simulink model "DriveTrain_SystemID3"  (R2019a)
settings: Solver=VariableStepAuto  StartTime=0.0  StopTime=20  MaxStep=1e-3  RelTol=1e-3
InitFcn:
  | %DriveTrainInitialise;
values from neighbouring files (symbols this model uses):
  D = 0.04925    [DrivetrainParametersForRhys.m]
  J = 0.0256    [DrivetrainParametersForRhys.m]
  Ld = 125e-6    (= 0.000125)    [DrivetrainParametersForRhys.m]
  Lq = 130e-6    (= 0.00013)    [DrivetrainParametersForRhys.m]
  p = PolePairs    (= 10)    [DrivetrainParametersForRhys.m]
  PM = 0.0393    [DrivetrainParametersForRhys.m]
  rate = 20    [DrivetrainParametersForRhys.m]
  ratio = 3.27    [DrivetrainParametersForRhys.m]
  Rs = 0.35    [DrivetrainParametersForRhys.m]
  Ts = 1/fs    (= 8.33333333333e-06)    [DrivetrainParametersForRhys.m]    (also in GreyBoxSystemID.m = mean(diff(posTime)))
  Tsc = 1/fc    (= 0.000166666666667)    [DrivetrainParametersForRhys.m]
  Vnom = 450    [DrivetrainParametersForRhys.m]
undefined symbols (not defined in the file or in its folder): Iq_max, Kaw, kdI, kdP, Ki, Kp, kqI, kqP
libraries: eeDqVoltageLimiter x1, eeTransforms x1
settings Model: OrderedModelArguments=off  Creator=plewi  LastModifiedBy=plewi

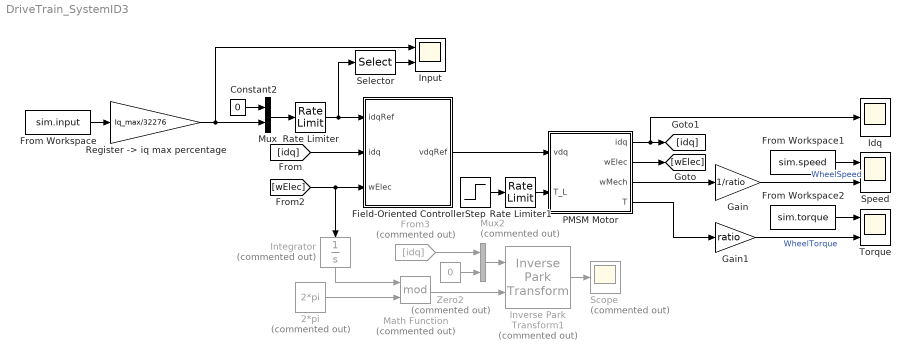
== system DriveTrain_SystemID3 ==
  2*pi : Constant  Commented=on  Value=2*pi  SampleTime=Tsc
  Constant2 : Constant  Value=0
  Field-Oriented Controller : Subsystem
  From Workspace : FromWorkspace  VariableName=sim.input  SampleTime=0
  From Workspace1 : FromWorkspace  VariableName=sim.speed  SampleTime=0
  From Workspace2 : FromWorkspace  VariableName=sim.torque  SampleTime=0
  From3 : From  Commented=on  GotoTag=idq
  Gain : Gain  Gain=1/ratio
  Gain1 : Gain  Gain=ratio
  Idq : Scope
  Input : Scope  NumInputPorts=2
  Integrator : Integrator  Commented=on
  Inverse Park Transform1 : eeTransforms/Inverse Park Transform  Commented=on  AxisAlignment=Q-axis  PowerInvariant=off
      settings: SourceProductName=Simscape Electrical
  Math Function : Math  Commented=on  Operator=mod  SaturateOnIntegerOverflow=on
  Mux : Mux  Inputs=2
  Mux2 : Mux  Commented=on  Inputs=2
  PMSM Motor : Subsystem
  Rate Limiter : RateLimiter  RisingSlewLimit=rate  FallingSlewLimit=-rate  SampleTimeMode=inherited
  Rate Limiter1 : RateLimiter  RisingSlewLimit=rate  FallingSlewLimit=-rate  SampleTimeMode=inherited
  "Register -> iq max percentage" : Gain  Gain=Iq_max/32276
  Scope : Scope  Commented=on
  Selector : Selector  InputPortWidth=2  IndexOptions=Index vector (dialog)  Indices=[2]  OutputSizes=1
  Speed : Scope  NumInputPorts=2
  Step : Step  Time=0  After=0  SampleTime=0
  Torque : Scope  NumInputPorts=2
  Zero2 : Constant  Commented=on  Value=0  OutDataTypeStr=Inherit: Inherit via back propagation
  wires:
  From Workspace/1 -> "Register -> iq max percentage"/1
  "Register -> iq max percentage"/1 -> Input/1, Mux/2
  Constant2/1 -> Mux/1
  From Workspace1/1 -> Speed/1
  From Workspace2/1 -> Torque/1
  Mux/1 -> Rate Limiter/1
  Rate Limiter/1 -> Selector/1, Field-Oriented Controller/1(idqRef)
  Selector/1 -> Input/2
  2*pi/1 -> Math Function/2
  Integrator/1 -> Math Function/1
  [wElec] -> Field-Oriented Controller/3(wElec), Integrator/1
  PMSM Motor/1("idq ") -> Idq/1, [idq]
  [idq] -> Field-Oriented Controller/2(idq)
  PMSM Motor/2(wElec) -> [wElec]
  Gain/1 -> Speed/2  "WheelSpeed"
  PMSM Motor/3(wMech) -> Gain/1
  PMSM Motor/4(T) -> Gain1/1
  Gain1/1 -> Torque/2  "WheelTorque"
  Math Function/1 -> Inverse Park Transform1/2
  Inverse Park Transform1/1 -> Scope/1
  Zero2/1 -> Mux2/2
  From3/1 -> Mux2/1
  Mux2/1 -> Inverse Park Transform1/1
  Field-Oriented Controller/1(vdqRef) -> PMSM Motor/1(vdq)
  Step/1 -> Rate Limiter1/1
  Rate Limiter1/1 -> PMSM Motor/2(T_L)

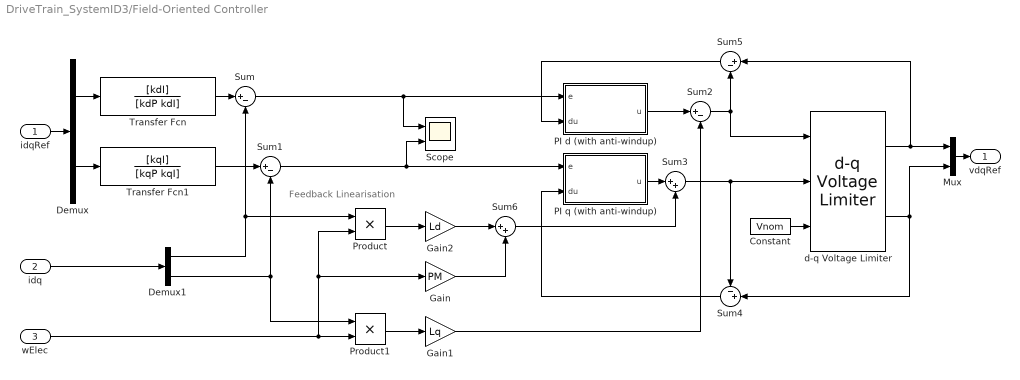
== system DriveTrain_SystemID3/Field-Oriented Controller ==
  note: Feedback Linearisation
  idqRef : Inport  SampleTime=Ts
  idq : Inport  Port=2  SampleTime=Ts
  wElec : Inport  Port=3  SampleTime=Ts
  Constant : Constant  Value=Vnom
  Demux : Demux  Outputs=2
  Demux1 : Demux  Outputs=2
  Gain : Gain  Gain=PM
  Gain1 : Gain  Gain=Lq
  Gain2 : Gain  Gain=Ld
  Mux : Mux  Inputs=2
  PI d (with anti-windup) : Subsystem
  PI q (with anti-windup) : Subsystem
  Product : Product
  Product1 : Product
  Scope : Scope  NumInputPorts=2
  Sum{,1..2,5} (4 alike) : Sum  Inputs=|+-
  Sum3 : Sum  Inputs=|++
  Sum4 : Sum  Inputs=-+|
  Sum6 : Sum  Inputs=|++
  Transfer Fcn : TransferFcn  Numerator=[kdI]  Denominator=[kdP kdI]
  Transfer Fcn1 : TransferFcn  Numerator=[kqI]  Denominator=[kqP kqI]
  d-q Voltage Limiter : eeDqVoltageLimiter/d-q Voltage Limiter  AxisPrio=Q-axis  Ts=-1
      settings: SourceProductName=Simscape Electrical  SourceProductBaseCode=PS
  vdqRef : Outport
  wires:
  Sum/1 -> Scope/1, PI d (with anti-windup)/1(e)
  Transfer Fcn1/1 -> Sum1/1
  Transfer Fcn/1 -> Sum/1
  d-q Voltage Limiter/2 -> Mux/2, Sum4/2
  idq/1 -> Demux1/1
  idqRef/1 -> Demux/1
  Sum2/1 -> d-q Voltage Limiter/1, Sum5/2
  Sum5/1 -> PI d (with anti-windup)/2(du)
  Demux/1 -> Transfer Fcn/1
  Constant/1 -> d-q Voltage Limiter/3
  Demux/2 -> Transfer Fcn1/1
  Sum3/1 -> d-q Voltage Limiter/2, Sum4/1
  d-q Voltage Limiter/1 -> Mux/1, Sum5/1
  Sum6/1 -> Sum3/2
  PI d (with anti-windup)/1(u) -> Sum2/1
  Sum4/1 -> PI q (with anti-windup)/2(du)
  Sum1/1 -> Scope/2, PI q (with anti-windup)/1(e)
  PI q (with anti-windup)/1(u) -> Sum3/1
  Demux1/1 -> Product/1, Sum/2
  Demux1/2 -> Sum1/2, Product1/1
  Gain/1 -> Sum6/2
  Product1/1 -> Gain1/1
  Gain1/1 -> Sum2/2
  Product/1 -> Gain2/1
  Gain2/1 -> Sum6/1
  wElec/1 -> Gain/1, Product/2, Product1/2
  Mux/1 -> vdqRef/1

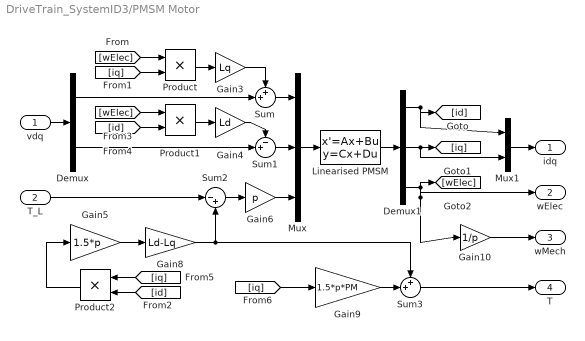
== system DriveTrain_SystemID3/PMSM Motor ==
  vdq : Inport
  T_L : Inport  Port=2
  Demux : Demux  Outputs=2
  Demux1 : Demux  Outputs=3
  Gain10 : Gain  Gain=1/p
  Gain3 : Gain  Gain=Lq
  Gain4 : Gain  Gain=Ld
  Gain5 : Gain  Gain=1.5*p
  Gain6 : Gain  Gain=p
  Gain8 : Gain  Gain=Ld-Lq
  Gain9 : Gain  Gain=1.5*p*PM
  "Linearised PMSM " : StateSpace  A=inv(diag([Ld,Lq,J]))*[-Rs, 0, 0; 0, -Rs, -PM; 0, 1.5*(p^2)*PM, -D]  B=inv(diag([Ld,Lq,J]))*eye(3)  C=eye(3)  D=zeros(3)  InitialCondition=0
  Mux : Mux  Inputs=3
  Mux1 : Mux  Inputs=2
  Product : Product
  Product1 : Product
  Product2 : Product
  Sum : Sum  Inputs=++|
  Sum1 : Sum  Inputs=-+|
  Sum2 : Sum  Inputs=|-+
  Sum3 : Sum  Inputs=++|
  "idq " : Outport
  wElec : Outport  Port=2
  wMech : Outport  Port=3
  T : Outport  Port=4
  wires:
  vdq/1 -> Demux/1
  "Linearised PMSM "/1 -> Demux1/1
  Demux1/1 -> Mux1/1, [id]
  Demux1/2 -> Mux1/2, [iq]
  Demux1/3 -> Gain10/1, wElec/1, [wElec]
  [wElec] -> Product/1
  [iq] -> Product/2
  Product/1 -> Gain3/1
  Gain3/1 -> Sum/1
  Demux/1 -> Sum/2
  Mux/1 -> "Linearised PMSM "/1
  Sum/1 -> Mux/1
  [id] -> Product1/2
  Product1/1 -> Gain4/1
  [wElec] -> Product1/1
  Sum1/1 -> Mux/2
  Gain4/1 -> Sum1/1
  Demux/2 -> Sum1/2
  [iq] -> Product2/1
  [id] -> Product2/2
  Product2/1 -> Gain5/1
  T_L/1 -> Sum2/1
  Sum2/1 -> Gain6/1
  Gain6/1 -> Mux/3
  [iq] -> Gain9/1
  Gain8/1 -> Sum3/1, Sum2/2
  Sum3/1 -> T/1
  Gain9/1 -> Sum3/2
  Gain10/1 -> wMech/1
  Mux1/1 -> "idq "/1
  Gain5/1 -> Gain8/1

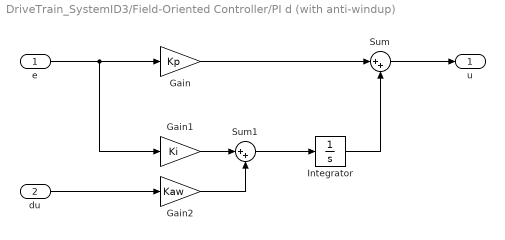
== system DriveTrain_SystemID3/Field-Oriented Controller/PI d (with anti-windup) ==
  e : Inport  SampleTime=Ts
  du : Inport  Port=2  SampleTime=Ts
  Gain : Gain  Gain=Kp
  Gain1 : Gain  Gain=Ki
  Gain2 : Gain  Gain=Kaw
  Integrator : Integrator
  Sum : Sum  Inputs=|++
  Sum1 : Sum  Inputs=|++
  u : Outport
  wires:
  e/1 -> Gain1/1, Gain/1
  Gain2/1 -> Sum1/2
  du/1 -> Gain2/1
  Sum1/1 -> Integrator/1
  Sum/1 -> u/1
  Integrator/1 -> Sum/2
  Gain1/1 -> Sum1/1
  Gain/1 -> Sum/1

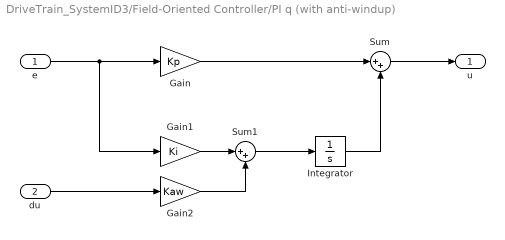
== system DriveTrain_SystemID3/Field-Oriented Controller/PI q (with anti-windup) ==
  e : Inport  SampleTime=Ts
  du : Inport  Port=2  SampleTime=Ts
  Gain : Gain  Gain=Kp
  Gain1 : Gain  Gain=Ki
  Gain2 : Gain  Gain=Kaw
  Integrator : Integrator
  Sum : Sum  Inputs=|++
  Sum1 : Sum  Inputs=|++
  u : Outport
  wires:
  e/1 -> Gain1/1, Gain/1
  Gain2/1 -> Sum1/2
  du/1 -> Gain2/1
  Sum1/1 -> Integrator/1
  Sum/1 -> u/1
  Integrator/1 -> Sum/2
  Gain1/1 -> Sum1/1
  Gain/1 -> Sum/1
